simulink model "Moore_Machine"  (R2020a)
settings: Solver=FixedStepDiscrete  StartTime=0.0  StopTime=150  FixedStep=0.1  RelTol=1e-3  EnableMultiTasking=on
undefined symbols (not defined in the file): DiscIntNeverNeededParam
libraries: simulink x1
settings Model: Creator=DELL  LastModifiedBy=DELL

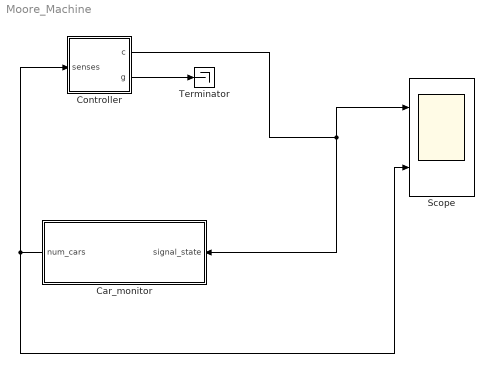
== system Moore_Machine ==
  Car_monitor : Subsystem
      settings: PortSchema="{\"entries\":[{\"content\":{\"sides\":[{\"content\":{\"connectorIds\":[\"Out1\"]},\"type\":\"ConnectorPlacement.EquallySpacedRectSide\",\"uuid\":\"bcbf8eaa-f28f-4157-93e4-f25bf0014ff7\"},{\"content\":{\"connectorIds\":[\"In1\"],\"side\":\"RIGHT\"},\"type\":\"ConnectorPlacement.EquallySpacedRectSide\",\"uuid\":\"3b56eafb-13f5-4690-ab3e-a10d29c7a0d5\"},{\"content\":{\"connectorIds\":[],\"side\":\"TOP\"},\"type\":\"ConnectorPlacement.EquallySpacedRectSide\",\"uuid\":\"bcfb9d30-9dc9-49f1-a40b-20ab5a5d93aa\"}]},\"type\":\"ConnectorPlacement.EquallySpacedConnector\",\"uuid\":\"c0706d9f-ec08-44c8-a295-a6a0464ad35f\"}],\"packageUris\":[\"http://schema.mathworks.com/mf0/Connector/19700101\"],\"version\":\"1.0\"}"
  Controller : Stateflow chart  TreatAsAtomicUnit=on
  Scope : Scope  NumInputPorts=2
  Terminator : Terminator
  wires:
  Controller/1(c) -> Car_monitor/1(signal_state), Scope/1
  Controller/2(g) -> Terminator/1
  Car_monitor/1(num_cars) -> Controller/1(senses), Scope/2

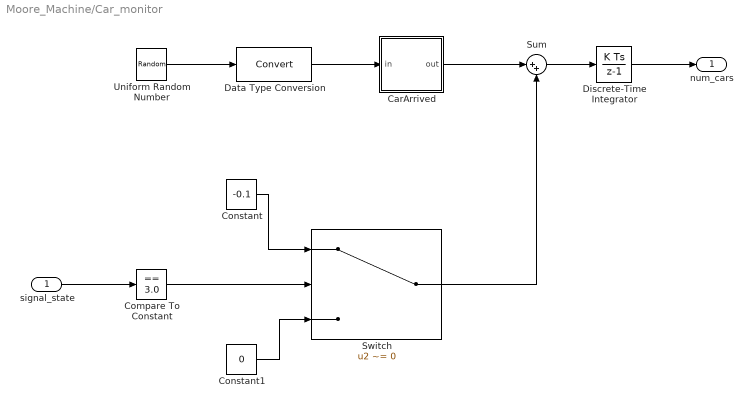
== system Moore_Machine/Car_monitor ==
  signal_state : Inport
  CarArrived : Stateflow chart  TreatAsAtomicUnit=on
  Compare To Constant : simulink/Logic and Bit Operations/Compare To Constant  relop===  const=3.0  OutDataTypeStr=boolean  ZeroCross=off
  Constant : Constant  Value=-0.1
  Constant1 : Constant  Value=0
  Data Type Conversion : DataTypeConversion
  Discrete-Time Integrator : DiscreteIntegrator  SampleTime=-1  LimitOutput=on  LowerSaturationLimit=0  ICPrevOutput=DiscIntNeverNeededParam  ICPrevScaledInput=DiscIntNeverNeededParam
  Sum : Sum  Inputs=|++
  Switch : Switch  Criteria=u2 ~= 0
  Uniform Random Number : UniformRandomNumber  Minimum=0  Maximum=100  Seed=177836  SampleTime=0
  num_cars : Outport
  wires:
  Constant/1 -> Switch/1
  signal_state/1 -> Compare To Constant/1
  Uniform Random Number/1 -> Data Type Conversion/1
  Sum/1 -> Discrete-Time Integrator/1
  Data Type Conversion/1 -> CarArrived/1(in)
  Switch/1 -> Sum/2
  Constant1/1 -> Switch/3
  CarArrived/1(out) -> Sum/1
  Compare To Constant/1 -> Switch/2
  Discrete-Time Integrator/1 -> num_cars/1

== stateflow chart Moore_Machine/Controller ==
  settings: stateMachineType=MOORE_MACHINE  initializeOutput=1
  state Stop
    c = Red;
    g = Green;
  state StopforTraffic
    c = Red;
    g = Green;
  state StopTogo
    c = Red;
    g = Yellow;
  state GotoStop
    c = Yellow;
    g = Red;
  state Go
    c = Green;
    g = Red;
  (default) -> Stop
  Stop -> StopforTraffic : after(20,tick)
  StopforTraffic -> StopTogo : [senses]
  GotoStop -> Stop : after(3,tick)
  StopTogo -> Go : after(3,tick)
  Go -> GotoStop : after(10,tick)
  data: c output; g output; Red constant double =1; Yellow constant double =2; Green constant double =3; senses input

== stateflow chart Moore_Machine/Car_monitor/CarArrived ==
  (default) -> (junction 1) : {out = in > 98;}
  data: in input; out output
